simulink model "PiekarekLabNr3_si"  (R2022b)
settings: Solver=VariableStepAuto  StartTime=0.0  StopTime=5000  MaxStep=5  RelTol=1e-3
values from neighbouring files (symbols this model uses):
  cpp = 1000    [PiekarekLabNr3.m]
  Cvp = cpp*rop*Vp    (= 6000)    [PiekarekLabNr3.m]
  Cvv = cpp*rop*Vw    (= 12000)    [PiekarekLabNr3.m]
  czas_skok = 5000    [PiekarekLabNr3.m]
  dFp = 0    [PiekarekLabNr3.m]
  dPg = 0    [PiekarekLabNr3.m]
  dTzew = 0    [PiekarekLabNr3.m]
  Fp0 = fPN    (= 0.000231481481481)    [PiekarekLabNr3.m]
  K1 = 2*Kd    (= 347.632850242)    [PiekarekLabNr3.m]
  Kd = (PgN-cpp*rop*fPN*(TwewN-TzewN))/(2*(TwewN-TzewN) +7*(TwewN-TpN))    (= 173.816425121)    [PiekarekLabNr3.m]
  Kp = (Kd*(TpN-TzewN))/(TwewN-TpN)    (= 1216.71497585)    [PiekarekLabNr3.m]
  PgN = 20000    [PiekarekLabNr3.m]
  rop = 1.2    [PiekarekLabNr3.m]
  Tp0 = (PgN+(Kd*K1*Tzew0)+(K1+Kp+Tzew0)+(cpp*rop*Fp0*Kd*Tzew0)+(cpp*rop*Fp0*Kp*Tzew0)+(Kd*Kp*Tzew0))/(K1+Kd+(cpp*rop*Fp0*Kd)-(Kd*Kp))    (= 25.7182260074)    [PiekarekLabNr3.m]
  Twew0 = Kd/Kp*(Tp0-Tzew0)+Tp0    (= 32.2494011513)    [PiekarekLabNr3.m]
  Tzew0 = TzewN    (= -20)    [PiekarekLabNr3.m]
settings Model: Creator=Lab320  LastModifiedBy=Lenovo
settings SolverCC: AlgebraicLoopSolver=TrustRegion
settings DebuggingCC: UnconnectedInputMsg=warning  UnconnectedOutputMsg=warning  UnconnectedLineMsg=warning  SFMachineParentedDataDiag=warning
settings ModelReferenceCC: EnableRefExpFcnMdlSchedulingChecks=on
settings RTWCC: DLArmComputeVersion=19.05

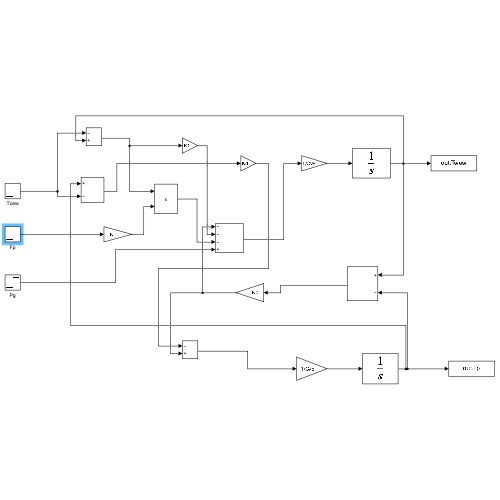
[thumbnail: Simulink's stored preview of the top-level diagram]
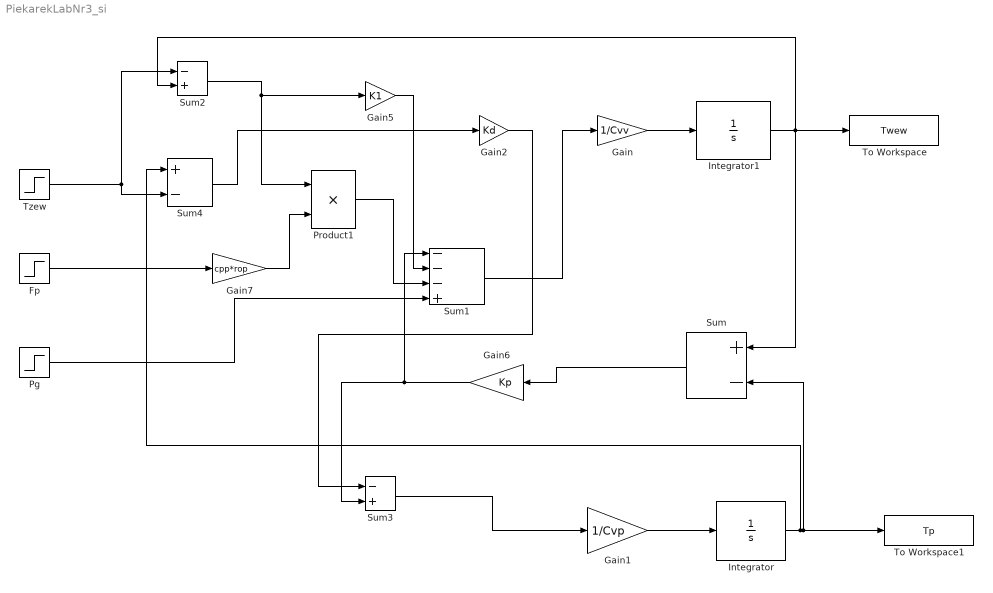
== system PiekarekLabNr3_si ==
  Fp : Step  Time=czas_skok  Before=Fp0  After=Fp0+dFp  SampleTime=0
  Gain : Gain  Gain=1/Cvv
  Gain1 : Gain  Gain=1/Cvp
  Gain2 : Gain  Gain=Kd
  Gain5 : Gain  Gain=K1
  Gain6 : Gain  Gain=Kp
  Gain7 : Gain  Gain=cpp*rop
  Integrator : Integrator  InitialCondition=Tp0
  Integrator1 : Integrator  InitialCondition=Twew0
  Pg : Step  Time=czas_skok  Before=PgN  After=PgN+dPg  SampleTime=0
  Product1 : Product
  Sum : Sum  Inputs=+-
  Sum1 : Sum  Inputs=---+
  Sum2 : Sum  Inputs=-+
  Sum3 : Sum  Inputs=-+
  Sum4 : Sum  Inputs=+-
  To Workspace : ToWorkspace  VariableName=Twew  SampleTime=-1
  To Workspace1 : ToWorkspace  VariableName=Tp  SampleTime=-1
  Tzew : Step  Time=czas_skok  Before=Tzew0  After=Tzew0+dTzew  SampleTime=0
  wires:
  Gain/1 -> Integrator1/1
  Gain1/1 -> Integrator/1
  Fp/1 -> Gain7/1
  Tzew/1 -> Sum4/2, Sum2/1
  Integrator1/1 -> Sum2/2, Sum/1, To Workspace/1
  Integrator/1 -> Sum4/1, Sum/2, To Workspace1/1
  Sum3/1 -> Gain1/1
  Gain7/1 -> Product1/2
  Sum2/1 -> Product1/1, Gain5/1
  Gain6/1 -> Sum1/1, Sum3/2
  Sum/1 -> Gain6/1
  Sum1/1 -> Gain/1
  Product1/1 -> Sum1/3
  Gain5/1 -> Sum1/2
  Sum4/1 -> Gain2/1
  Pg/1 -> Sum1/4
  Gain2/1 -> Sum3/1
